simulink model "simulate_drone"  (R2021a)
settings: Solver=VariableStepAuto  StartTime=0.0  StopTime=120.0  RelTol=1e-3
PreLoadFcn:
  | init;
undefined symbols (not defined in the file or in its folder): Param
settings Model: Creator=Bruno  LastModifiedBy=Nunes
settings SolverCC: AlgebraicLoopSolver=TrustRegion
settings DebuggingCC: SFMachineParentedDataDiag=warning

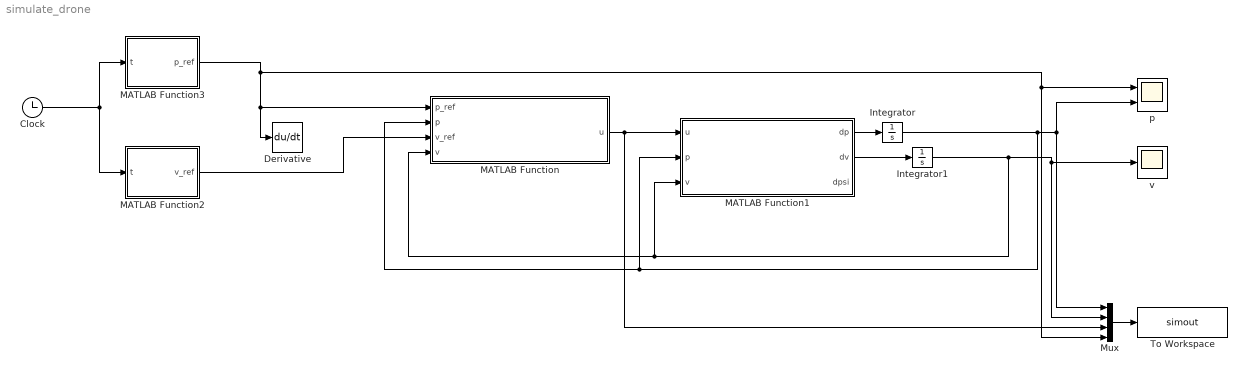
== system simulate_drone ==
  Clock : Clock
  Derivative : Derivative
  Integrator : Integrator  InitialCondition=Param.p0
  Integrator1 : Integrator  InitialCondition=Param.v0
  MATLAB Function : MATLAB Function  TreatAsAtomicUnit=on
  MATLAB Function1 : MATLAB Function  TreatAsAtomicUnit=on
  MATLAB Function2 : MATLAB Function  TreatAsAtomicUnit=on
  MATLAB Function3 : MATLAB Function  TreatAsAtomicUnit=on
  Mux : Mux
  To Workspace : ToWorkspace  VariableName=simout  SaveFormat=Timeseries  SampleTime=-1
  p : Scope  NumInputPorts=2
  "v " : Scope
  wires:
  MATLAB Function/1(u) -> MATLAB Function1/1(u), Mux/3
  MATLAB Function1/1(dp) -> Integrator/1
  MATLAB Function1/2(dv) -> Integrator1/1
  Integrator/1 -> p/2, Mux/1, MATLAB Function1/2(p), MATLAB Function/2(p)
  Integrator1/1 -> Mux/2, "v "/1, MATLAB Function/4(v), MATLAB Function1/3(v)
  Mux/1 -> To Workspace/1
  Clock/1 -> MATLAB Function3/1(t), MATLAB Function2/1(t)
  MATLAB Function3/1(p_ref) -> Mux/4, p/1, Derivative/1, MATLAB Function/1(p_ref)
  MATLAB Function2/1(v_ref) -> MATLAB Function/3(v_ref)

== matlab function simulate_drone/MATLAB Function1 ==
  data: u input; p input; v input; dp output; dv output; Param parameter; dpsi output
function [dp,dv,dpsi] = drone_model(u,p,v,Param)
%DRONE_MODEL Summary of this function goes here
%   Detailed explanation goes here

    P = Param;
    
    dp = v;
    dv = -[0;0;P.g] + 1/P.m*u;
    dpsi = 0;
    
end

== matlab function simulate_drone/MATLAB Function ==
  data: p_ref input; p input; v_ref input; u output; v input; Param parameter
function u = drone_controller(p_ref,p,v_ref,v,Param)
%DRONE_CONTROLLER Summary of this function goes here
%   Detailed explanation goes here

    P = Param;
    
    u = -diag([P.kp/2,P.kp/2,P.kp])*(p-p_ref) + ...
        -diag([P.kv/2,P.kv/2,P.kv])*(v-v_ref) + [0;0;P.m*P.g];
    
end

== matlab function simulate_drone/MATLAB Function2 ==
  data: t input; v_ref output

function v_ref = velocity_ref(t)





      
if t < 20
   v_ref = [ 1/2; 0 ; 0];
   
elseif t > 20 & t < 80 

   v_ref = [ 0; 0 ;0 ];
 
elseif t > 80 & t < 100 

   v_ref = [  - 1/2; 0 ;0 ];
else
     v_ref = [0;0;0];     
     
end





end


%plot da trajectoria -  plot3(out.simout.Data(:,1), out.simout.Data(:,2), out.simout.Data(:,3));

== matlab function simulate_drone/MATLAB Function3 ==
  data: t input; p_ref output

function p_ref = position_ref(t)


% if t < 30
%    p_ref = [sin(t);cos(t);3];
% else 
%     p_ref = [sin(t);cos(t);1];
% end



      
% if t < 20
%    p_ref = [1 + t/2; 1 ; 2];
%    
% elseif t > 20 & t < 40 
%    p_ref = [11+ cos(t) ; 2 + sin(t)  ;2 ];
%    %p_ref = [11 + cos(t); 2 +sin(t) ;2 ];
%    
% elseif t > 40 & t < 60 
%    p_ref = [ - t/2; 3 ;2 ];
%     
% else
%      p_ref = [0;0;0];     
%      
% end


      
if t < 20
   p_ref = [ t/2; 0 ; 0.5];
   
elseif t > 20 & t < 80 

   p_ref = [ 10; 2 ; 0.5];
   
    
elseif t > 80 & t < 100 

   p_ref = [ 50 - t/2; 2 ;0.5 ];
else
     p_ref = [0;0;0.5];     
     
end





end


%plot da trajectoria -  plot3(out.simout.Data(:,1), out.simout.Data(:,2), out.simout.Data(:,3));
